simulink model "nonlinear_quad_plant"  (R2019b)
settings: Solver=FixedStepAuto  StartTime=0.0  StopTime=200  FixedStep=5/1000  RelTol=1e-3
undefined symbols (not defined in the file or in its folder): DiscIntNeverNeededParam
libraries: simulink x4
settings Model: Creator=jarro  LastModifiedBy=jarro

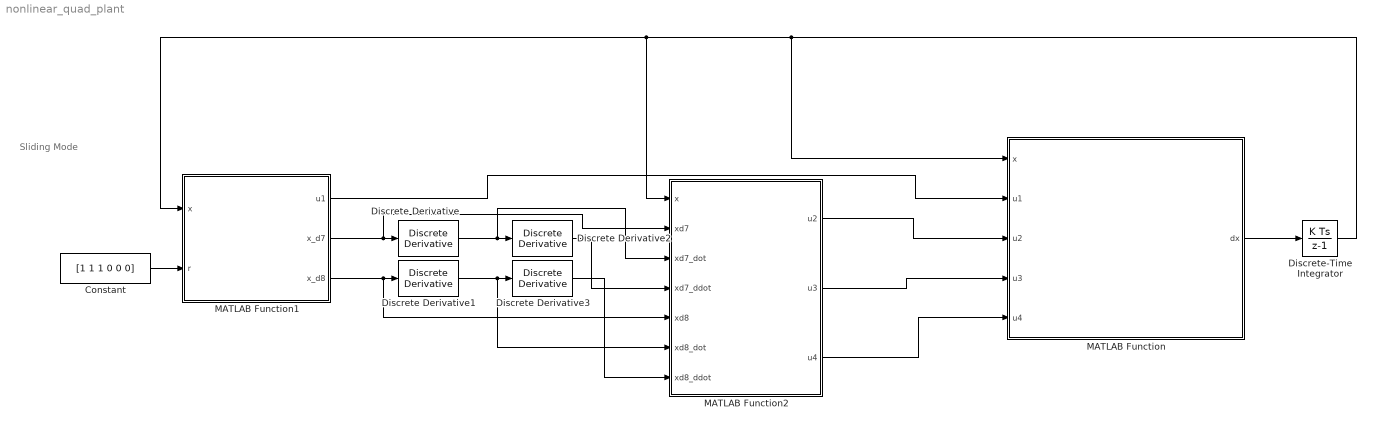
== system nonlinear_quad_plant ==
  note: Sliding Mode
  Constant : Constant  Value=[1 1 1 0 0 0]  SampleTime=5/1000
  Discrete Derivative{,1..3} (4 alike) : simulink/Discrete/Discrete Derivative  gainval=1.0  ICPrevScaledInput=0.0  OutMin=[]  OutMax=[]  OutDataType=fixdt(1, 16)  OutScaling=2^-10  DoSatur=off
  Discrete-Time Integrator : DiscreteIntegrator  InitialCondition=0.1*ones(12,1)  SampleTime=-1  ICPrevOutput=DiscIntNeverNeededParam  ICPrevScaledInput=DiscIntNeverNeededParam
  MATLAB Function : MATLAB Function  TreatAsAtomicUnit=on
  MATLAB Function1 : MATLAB Function  TreatAsAtomicUnit=on
  MATLAB Function2 : MATLAB Function  TreatAsAtomicUnit=on
  wires:
  MATLAB Function/1(dx) -> Discrete-Time Integrator/1
  Discrete-Time Integrator/1 -> MATLAB Function/1(x), MATLAB Function2/1(x), MATLAB Function1/1(x)
  MATLAB Function1/2(x_d7) -> MATLAB Function2/2(xd7), Discrete Derivative/1
  MATLAB Function1/3(x_d8) -> MATLAB Function2/5(xd8), Discrete Derivative1/1
  Discrete Derivative/1 -> MATLAB Function2/3(xd7_dot), Discrete Derivative2/1
  Discrete Derivative1/1 -> MATLAB Function2/6(xd8_dot), Discrete Derivative3/1
  MATLAB Function1/1(u1) -> MATLAB Function/2(u1)
  MATLAB Function2/1(u2) -> MATLAB Function/3(u2)
  MATLAB Function2/2(u3) -> MATLAB Function/4(u3)
  MATLAB Function2/3(u4) -> MATLAB Function/5(u4)
  Discrete Derivative2/1 -> MATLAB Function2/4(xd7_ddot)
  Discrete Derivative3/1 -> MATLAB Function2/7(xd8_ddot)
  Constant/1 -> MATLAB Function1/2(r)

== matlab function nonlinear_quad_plant/MATLAB Function1 ==
  data: x input; u1 output; r input; x_d7 output; x_d8 output
function [u1,x_d7,x_d8] = sliding_mode(x, r)

c1 = 1;
k1 = 0.1;
k2 = 0.1;

c_1 = 30;
k_1 = 5;
k_2 = 5;


m = 0.6;
g = 9.8;
Ix = 0.0092;
Iy = 0.0092;
Iz = 0.0101;

s1 = (r(6)-x(6)) + c_1*(r(3)-x(3));
sx = (r(4)-x(4)) + c1*(r(1)-x(1));
sy = (r(5)-x(5)) + c1*(r(2)-x(2));

u1 = -(m/(cos(x(7))*cos(x(8))))*(k_1*sign(s1)+k_2*s1+g+c1*(r(6)-x(6)));

ux = (m/u1)*(k1*sign(sx) + k2*sx + c1*(r(4)-x(4)));
uy = (m/u1)*(k1*sign(sy) + k2*sy + c1*(r(5)-x(5)));

x_d7 = (asin(-uy-floor(-uy))) + pi/2*floor(-uy); % desired as functions 
x_d8 = (asin(ux/cos(x_d7) - floor(ux/cos(x_d7))))+ pi/2*floor(ux/cos(x_d7));

== matlab function nonlinear_quad_plant/MATLAB Function ==
  settings: sampleTime=5/1000
  data: dx output size=12; x input size=12; u1 input size=1; u2 input size=1; u3 input; u4 input size=1
function dx = nonlinear_quad_plant(x, u1, u2, u3, u4)

g = 9.81;
Ix = 0.0092;
Iy = 0.0092;
Iz = 0.0101;
m = 0.6;
g = 9.8;

dx = zeros(12,1);
drag = 0.01;
dx(1) = x(4); 
dx(2) = x(5);
dx(3) = x(6);
dx(4) = cos(x(7))*sin(x(8))*(u1/m);
dx(5) = -sin(x(7))*(u1/m);
dx(6) = g - cos(x(7))*cos(x(8))*(u1/m);
dx(7) = x(10);
dx(8) = x(11);
dx(9) = x(12);
dx(10) = u2/Ix;
dx(11) = u3/Iy;
dx(12) = u4/Iz;

%dx = dx';
end

== matlab function nonlinear_quad_plant/MATLAB Function2 ==
  data: x input; xd7 input; xd7_dot input; xd7_ddot input; xd8 input; u2 output; u3 output; u4 output; xd8_dot input; xd8_ddot input
function [u2, u3, u4] = sliding_mode2(x, xd7,xd7_dot, xd7_ddot, xd8, xd8_dot, xd8_ddot)

k1 = 0.1;
k2 = 0.1;
c1 = 1;

Ix = 0.0092;
Iy = 0.0092;
Iz = 0.0101;

s2 = (xd7_dot-x(10)) + c1*(xd7-x(7));
s3 = (xd8_dot-x(11)) + c1*(xd8-x(8));
s4 = (0-x(12)) + c1*(0-x(9));
u2 = Ix*(k1*sign(s2)+k2*s2 + xd7_ddot + c1*(xd7_dot -x(10)));
u3 = Ix*(k1*sign(s3)+k2*s3 + xd8_ddot + c1*(xd8_dot -x(11)));
u4 = Ix*(k1*sign(s4)+k2*s4 + c1*(0 -x(12)));
